simulink model "PASTd_Amin"  (R2024b)
settings: Solver=VariableStepAuto  StartTime=0.0  StopTime=100  RelTol=1e-3
libraries: dspsrcs4 x1
settings Model: PauseTimes=0.01  Creator=keshm  LastModifiedBy=keshm

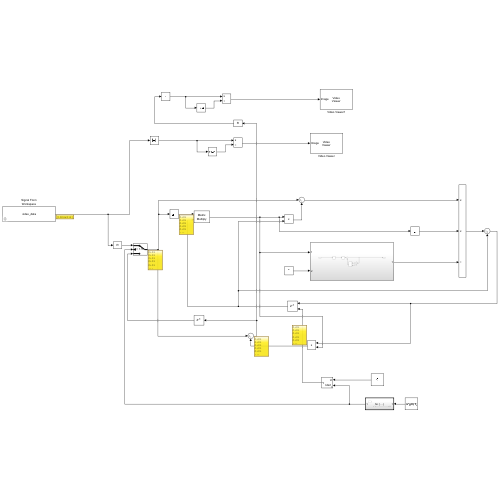
[thumbnail: Simulink's stored preview of the top-level diagram]
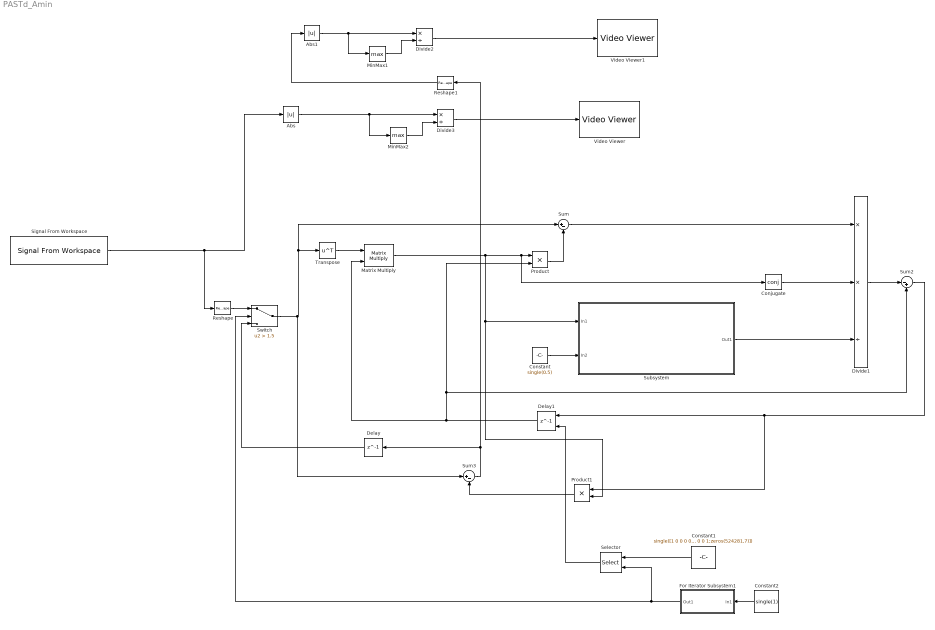
== system PASTd_Amin ==
  Abs : Abs  SaturateOnIntegerOverflow=off
  Abs1 : Abs  SaturateOnIntegerOverflow=off
  Conjugate : Math  Operator=conj  SignedPower=on  RndMeth=Zero
  Constant : Constant  Value=single(0.5)
  Constant1 : Constant  Value=single([1 0 0 0 0 0 0;0 1 0 0 0 0 0;0 0 1 0 0 0 0;0 0 0 1 0 0 0; 0 0 0 0 1 0 0; 0 0 0 0 0 1 0; 0 0 0 0 0 0 1;zeros(524281,7)])
  Constant2 : Constant  Value=single(1)
  Delay : Delay  DelayLength=1  InitialCondition=0
  Delay1 : Delay  DelayLength=1  InitialConditionSource=Input port  InitialCondition=0
      settings: InputPortMap=u0,p4
  Divide1 : Product  Inputs=**/
  Divide2 : Product  Inputs=*/
  Divide3 : Product  Inputs=*/
  For Iterator Subsystem1 : Subsystem  TreatAsAtomicUnit=on
  Matrix Multiply : Product  Multiplication=Matrix(*)
  MinMax1 : MinMax  Function=max
  MinMax2 : MinMax  Function=max
  Product : Product
  Product1 : Product
  Reshape : Reshape  OutputDimensionality=Customize  OutputDimensions=[524288,1]
  Reshape1 : Reshape  OutputDimensionality=Customize  OutputDimensions=[1024,512]
  Selector : Selector  NumberOfDimensions=2  InputPortWidth=3  IndexOptions=Select all,Index vector (port)  Indices=[1 3],1  OutputSizes=1,1
  Signal From Workspace : dspsrcs4/Signal From Workspace  X=video_data  Ts=1  nsamps=1  OutputAfterFinalValue=Setting to zero  ignoreOrWarnInputAndFrameLengths=off  OutputFrames=off
  Subsystem : Subsystem
  Sum : Sum  Inputs=|+-
  Sum2 : Sum  Inputs=|-+
  Sum3 : Sum  Inputs=|+-
  Switch : Switch  Criteria=u2 > Threshold  Threshold=1.5  SaturateOnIntegerOverflow=off  InputSameDT=off
  Transpose : Math  Operator=transpose
  Video Viewer : VideoViewer  FigPos=[765.8 818.8 766.4 708]
  Video Viewer1 : VideoViewer  FigPos=[30.6 817.2 766.4 708]
  wires:
  Signal From Workspace/1 -> Reshape/1, Abs/1
  Matrix Multiply/1 -> Product1/2, Subsystem/1(In1), Conjugate/1, Product/1
  Sum2/1 -> Product1/1, Delay1/1
  Product1/1 -> Sum3/2
  Subsystem/1(Out1) -> Divide1/3
  Sum/1 -> Divide1/1
  Conjugate/1 -> Divide1/2
  Product/1 -> Sum/2
  Divide1/1 -> Sum2/1
  Constant/1 -> Subsystem/2(In2)
  Constant1/1 -> Selector/1
  For Iterator Subsystem1/1(Out1) -> Switch/2, Selector/2
  Selector/1 -> Delay1/2
  Sum3/1 -> Reshape1/1, Delay/1
  MinMax1/1 -> Divide2/2
  Divide2/1 -> Video Viewer1/1
  Abs1/1 -> Divide2/1, MinMax1/1
  Reshape1/1 -> Abs1/1
  Delay1/1 -> Matrix Multiply/2, Sum2/2, Product/2
  Transpose/1 -> Matrix Multiply/1
  Reshape/1 -> Switch/1
  Switch/1 -> Sum3/1, Sum/1, Transpose/1
  Delay/1 -> Switch/3
  Constant2/1 -> For Iterator Subsystem1/1(In1)
  MinMax2/1 -> Divide3/2
  Abs/1 -> Divide3/1, MinMax2/1
  Divide3/1 -> Video Viewer/1

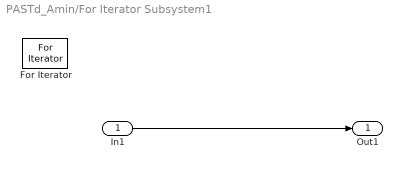
== system PASTd_Amin/For Iterator Subsystem1 ==
  In1 : Inport
  For Iterator : ForIterator  IterationLimit=2
  Out1 : Outport
  wires:
  In1/1 -> Out1/1

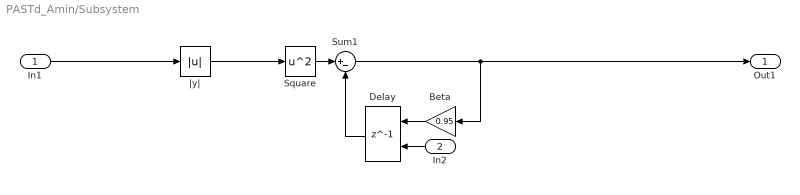
== system PASTd_Amin/Subsystem ==
  In1 : Inport
  In2 : Inport  Port=2
  Beta : Gain  Gain=0.95
  Delay : Delay  DelayLength=1  InitialConditionSource=Input port  InitialCondition=0
      settings: InputPortMap=u0,p4
  Square : Math  Operator=square
  Sum1 : Sum  Inputs=|+-
  |y| : Abs  SaturateOnIntegerOverflow=off
  Out1 : Outport
  wires:
  Square/1 -> Sum1/1
  Sum1/1 -> Out1/1, Beta/1
  Delay/1 -> Sum1/2
  In1/1 -> |y|/1
  Beta/1 -> Delay/1
  |y|/1 -> Square/1
  In2/1 -> Delay/2
